simulink model "Asw_PMSMCtrl"  (R2023a)
settings: Solver=FixedStepDiscrete  StartTime=0.0  StopTime=10.0  RelTol=1e-3
values from neighbouring files (symbols this model uses):
  Mt_Par_fNp = Simulink.Parameter    [Asw_PMSMCtrl_Parameters.m]
undefined symbols (not defined in the file or in its folder): Sw_Par_fTs
settings Model: Creator=62555  LastModifiedBy=62555

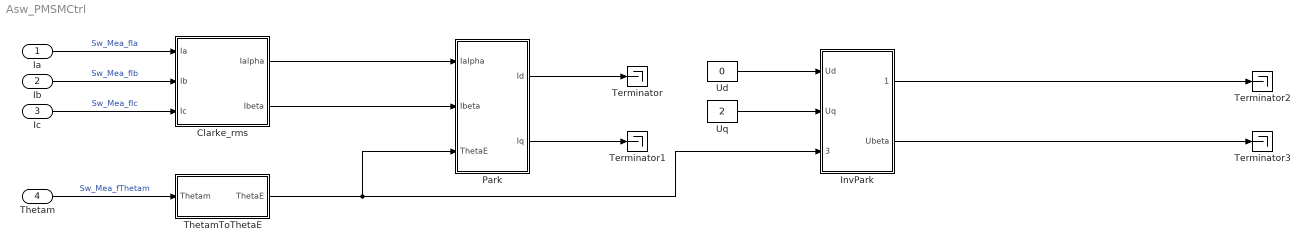
== system Asw_PMSMCtrl ==
  Ia : Inport
  Ib : Inport  Port=2
  Ic : Inport  Port=3
  Thetam : Inport  Port=4
  Clarke_rms : Subsystem
  InvPark : Subsystem
  Park : Subsystem
  Terminator{,1..3} (4 alike) : Terminator
  ThetamToThetaE : Subsystem
  Ud : Constant  Value=0  OutDataTypeStr=single  SampleTime=Sw_Par_fTs
  Uq : Constant  Value=2  OutDataTypeStr=single  SampleTime=Sw_Par_fTs
  wires:
  Clarke_rms/2(Ibeta) -> Park/2(Ibeta)
  InvPark/1(Ualpha) -> Terminator2/1
  Ud/1 -> InvPark/1(Ud)
  Uq/1 -> InvPark/2(Uq)
  Clarke_rms/1(Ialpha) -> Park/1(Ialpha)
  Ia/1 -> Clarke_rms/1(Ia)  "Sw_Mea_fIa"
  Ib/1 -> Clarke_rms/2(Ib)  "Sw_Mea_fIb"
  ThetamToThetaE/1(ThetaE) -> InvPark/3(ThetaE), Park/3(ThetaE)
  InvPark/2(Ubeta) -> Terminator3/1
  Ic/1 -> Clarke_rms/3(Ic)  "Sw_Mea_fIc"
  Park/2(Iq) -> Terminator1/1
  Park/1(Id) -> Terminator/1
  Thetam/1 -> ThetamToThetaE/1(Thetam)  "Sw_Mea_fThetam"

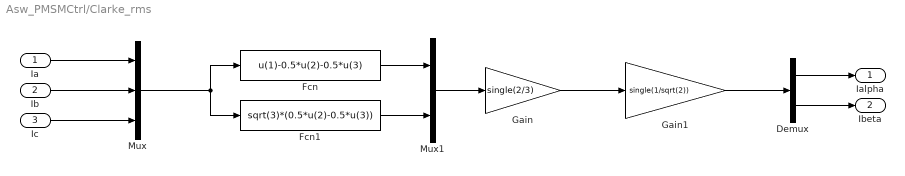
== system Asw_PMSMCtrl/Clarke_rms ==
  Ia : Inport
  Ib : Inport  Port=2
  Ic : Inport  Port=3
  Demux : Demux  Outputs=2
  Fcn : Fcn  Expr=u(1)-0.5*u(2)-0.5*u(3)
  Fcn1 : Fcn  Expr=sqrt(3)*(0.5*u(2)-0.5*u(3))
  Gain : Gain  Gain=single(2/3)
  Gain1 : Gain  Gain=single(1/sqrt(2))
  Mux : Mux  Inputs=3
  Mux1 : Mux  Inputs=2
  Ialpha : Outport
  Ibeta : Outport  Port=2
  wires:
  Gain1/1 -> Demux/1
  Mux/1 -> Fcn1/1, Fcn/1
  Mux1/1 -> Gain/1
  Fcn/1 -> Mux1/1
  Fcn1/1 -> Mux1/2
  Gain/1 -> Gain1/1
  Ia/1 -> Mux/1
  Ib/1 -> Mux/2
  Ic/1 -> Mux/3
  Demux/1 -> Ialpha/1
  Demux/2 -> Ibeta/1

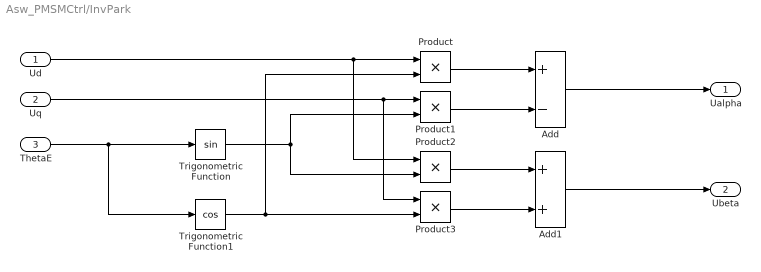
== system Asw_PMSMCtrl/InvPark ==
  Ud : Inport
  Uq : Inport  Port=2
  ThetaE : Inport  Port=3
  Add : Sum  Inputs=+-
  Add1 : Sum
  Product{,1..3} (4 alike) : Product
  Trigonometric Function : Trigonometry
  Trigonometric Function1 : Trigonometry  Operator=cos
  Ualpha : Outport
  Ubeta : Outport  Port=2
  wires:
  Ud/1 -> Product2/1, Product/1
  ThetaE/1 -> Trigonometric Function1/1, Trigonometric Function/1
  Uq/1 -> Product3/1, Product1/1
  Trigonometric Function/1 -> Product2/2, Product1/2
  Product1/1 -> Add/2
  Trigonometric Function1/1 -> Product/2, Product3/2
  Product/1 -> Add/1
  Product3/1 -> Add1/2
  Add/1 -> Ualpha/1
  Product2/1 -> Add1/1
  Add1/1 -> Ubeta/1

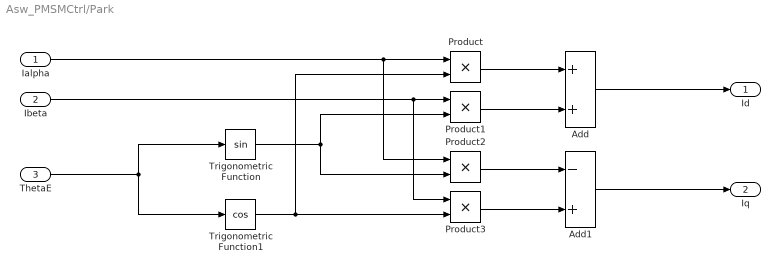
== system Asw_PMSMCtrl/Park ==
  Ialpha : Inport
  Ibeta : Inport  Port=2
  ThetaE : Inport  Port=3
  Add : Sum
  Add1 : Sum  Inputs=-+
  Product{,1..3} (4 alike) : Product
  Trigonometric Function : Trigonometry
  Trigonometric Function1 : Trigonometry  Operator=cos
  Id : Outport
  Iq : Outport  Port=2
  wires:
  Ibeta/1 -> Product3/1, Product1/1
  Product3/1 -> Add1/2
  ThetaE/1 -> Trigonometric Function1/1, Trigonometric Function/1
  Trigonometric Function/1 -> Product2/2, Product1/2
  Trigonometric Function1/1 -> Product/2, Product3/2
  Product2/1 -> Add1/1
  Product1/1 -> Add/2
  Product/1 -> Add/1
  Ialpha/1 -> Product2/1, Product/1
  Add/1 -> Id/1
  Add1/1 -> Iq/1

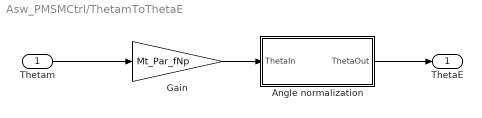
== system Asw_PMSMCtrl/ThetamToThetaE ==
  Thetam : Inport
  Angle normalization : MATLAB Function  TreatAsAtomicUnit=on
  Gain : Gain  Gain=Mt_Par_fNp
  ThetaE : Outport
  wires:
  Gain/1 -> Angle normalization/1(ThetaIn)
  Thetam/1 -> Gain/1
  Angle normalization/1(ThetaOut) -> ThetaE/1

== matlab function Asw_PMSMCtrl/ThetamToThetaE/Angle normalization ==
  data: ThetaIn input; ThetaOut output
function ThetaOut = fcn(ThetaIn)

Theta = ThetaIn;

while(Theta > 2*pi)
    Theta = Theta - 2*pi;
end

while(Theta < 0)
    Theta = Theta + 2*pi;
end

ThetaOut = Theta;
